simulink model "bmgen_array_N8"  (R2014a)
settings: Solver=ode45  StartTime=0.0  StopTime=Tmax  RelTol=1e-3
values from neighbouring files (symbols this model uses):
  Tgrid = (1 / Fgrid)    (= 0.0166666666667)    [array_init.m]
  Ts = Tthd    (= 1.66666666667e-05)    [array_init.m]
  Tstartup = 3e-3    (= 0.003)    [array_init.m]
  Vgrid = (sqrt(2)*Vgridrms)    [array_init.m]
undefined symbols (not defined in the file or in its folder): Acarray, Aoarray, Bcarray, Boarray, Carray, Darray, Larray, N, Rarray, TswitchArray
libraries: module_switch x8, powerlib_meascontrol x3
settings Model: Creator=Taylor  LastModifiedBy=Taylor

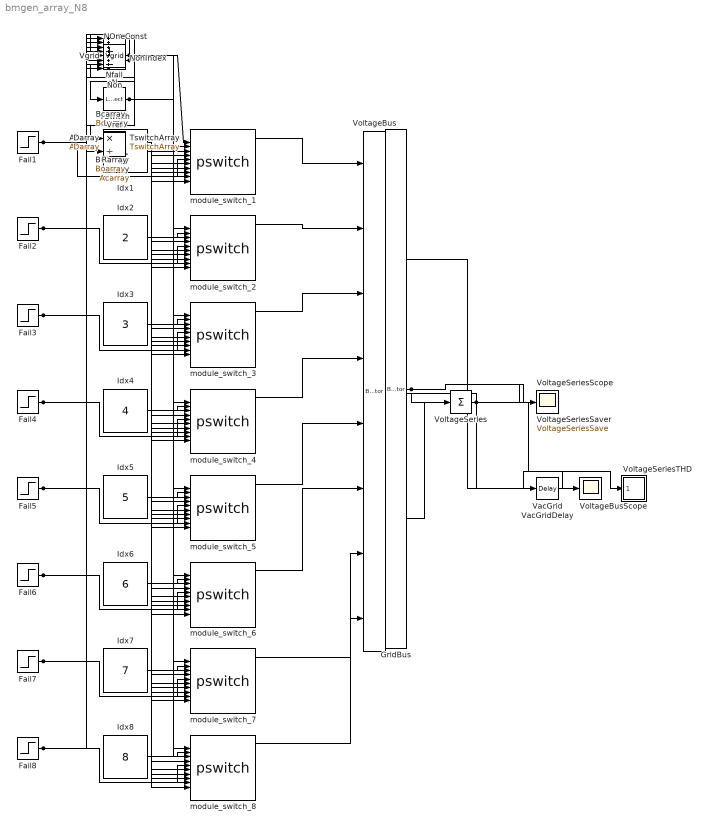
== system bmgen_array_N8 ==
  Acarray : Constant  Value=Acarray
  Aoarray : Constant  Value=Aoarray
  Bcarray : Constant  Value=Bcarray
  Boarray : Constant  Value=Boarray
  Carray : Constant  Value=Carray
  Darray : Constant  Value=Darray
  Fail{1..8} (8 alike) : Step  Time=0  After=0
  GridBus : BusCreator  Inputs=2
  Idx1 : Constant
  Idx2 : Constant  Value=2
  Idx3 : Constant  Value=3
  Idx4 : Constant  Value=4
  Idx5 : Constant  Value=5
  Idx6 : Constant  Value=6
  Idx7 : Constant  Value=7
  Idx8 : Constant  Value=8
  Larray : Constant  Value=Larray
  N : Constant  Value=N
  NOneConst : Constant
  Nfail : Sum  Inputs=++++++++  SaturateOnIntegerOverflow=on  InputSameDT=on  OutDataTypeStr=Inherit: Same as first input
  Non : Sum  Inputs=+-  SaturateOnIntegerOverflow=on  InputSameDT=on  OutDataTypeStr=Inherit: Same as first input
  NonIndex : Sum  Inputs=+-  SaturateOnIntegerOverflow=on  InputSameDT=on  OutDataTypeStr=Inherit: Same as first input
  Rarray : Constant  Value=Rarray
  TSwitch : LookupNDDirect  NumberOfTableDimensions=3  InputsSelectThisObjectFromTable=2-D Matrix  Table=TswitchArray
  TswitchArray : Constant  Value=TswitchArray
  VacGrid : Sin  Amplitude=Vgrid  Frequency=2*pi/Tgrid
  VacGridDelay : TransportDelay  DelayTime=Tstartup
  Vgrid : Constant  Value=Vgrid
  VoltageBus : BusCreator  Inputs=N
  VoltageBusScope : Scope
  VoltageSeries : Sum  Inputs=+  SaturateOnIntegerOverflow=on  InputSameDT=on  OutDataTypeStr=Inherit: Same as first input
  VoltageSeriesSaver : ToWorkspace  VariableName=VoltageSeriesSave
  VoltageSeriesScope : Scope
      settings: SaveName=ScopeDataSeries
  VoltageSeriesTHD : Subsystem  VariantControl=Variant1
  Vref : Product  Inputs=*/  SaturateOnIntegerOverflow=on  RndMeth=Zero  InputSameDT=on  OutDataTypeStr=Inherit: Same as first input
  module_switch_{1..8} (8 alike) : module_switch/pswitch
  wires:
  VacGrid/1 -> VacGridDelay/1
  VacGridDelay/1 -> GridBus/1
  N/1 -> Non/1, module_switch_1/1, module_switch_2/1, module_switch_3/1, module_switch_4/1, module_switch_5/1, module_switch_6/1, module_switch_7/1, module_switch_8/1
  Nfail/1 -> Non/2
  Non/1 -> NonIndex/1, Vref/2
  NOneConst/1 -> NonIndex/2
  Vgrid/1 -> Vref/1
  NonIndex/1 -> TSwitch/1
  VoltageSeries/1 -> GridBus/2, VoltageSeriesTHD/1(In1)
  VoltageBus/1 -> VoltageSeries/1, VoltageBusScope/1
  GridBus/1 -> VoltageSeriesScope/1, VoltageSeriesSaver/1
  Idx1/1 -> module_switch_1/2
  Fail1/1 -> module_switch_1/5, Nfail/1
  TSwitch/1 -> module_switch_1/3, module_switch_2/3, module_switch_3/3, module_switch_4/3, module_switch_5/3, module_switch_6/3, module_switch_7/3, module_switch_8/3
  Darray/1 -> module_switch_1/4, module_switch_2/4, module_switch_3/4, module_switch_4/4, module_switch_5/4, module_switch_6/4, module_switch_7/4, module_switch_8/4
  Acarray/1 -> module_switch_1/6, module_switch_2/6, module_switch_3/6, module_switch_4/6, module_switch_5/6, module_switch_6/6, module_switch_7/6, module_switch_8/6
  Aoarray/1 -> module_switch_1/7, module_switch_2/7, module_switch_3/7, module_switch_4/7, module_switch_5/7, module_switch_6/7, module_switch_7/7, module_switch_8/7
  Bcarray/1 -> module_switch_1/9, module_switch_2/9, module_switch_3/9, module_switch_4/9, module_switch_5/9, module_switch_6/9, module_switch_7/9, module_switch_8/9
  Boarray/1 -> module_switch_1/8, module_switch_2/8, module_switch_3/8, module_switch_4/8, module_switch_5/8, module_switch_6/8, module_switch_7/8, module_switch_8/8
  Vref/1 -> module_switch_1/10, module_switch_2/10, module_switch_3/10, module_switch_4/10, module_switch_5/10, module_switch_6/10, module_switch_7/10, module_switch_8/10
  module_switch_1/1 -> VoltageBus/1
  Idx2/1 -> module_switch_2/2
  Fail2/1 -> module_switch_2/5, Nfail/2
  module_switch_2/1 -> VoltageBus/2
  Idx3/1 -> module_switch_3/2
  Fail3/1 -> module_switch_3/5, Nfail/3
  module_switch_3/1 -> VoltageBus/3
  Idx4/1 -> module_switch_4/2
  Fail4/1 -> module_switch_4/5, Nfail/4
  module_switch_4/1 -> VoltageBus/4
  Idx5/1 -> module_switch_5/2
  Fail5/1 -> module_switch_5/5, Nfail/5
  module_switch_5/1 -> VoltageBus/5
  Idx6/1 -> module_switch_6/2
  Fail6/1 -> module_switch_6/5, Nfail/6
  module_switch_6/1 -> VoltageBus/6
  Idx7/1 -> module_switch_7/2
  Fail7/1 -> module_switch_7/5, Nfail/7
  module_switch_7/1 -> VoltageBus/7
  Idx8/1 -> module_switch_8/2
  Fail8/1 -> module_switch_8/5, Nfail/8
  module_switch_8/1 -> VoltageBus/8

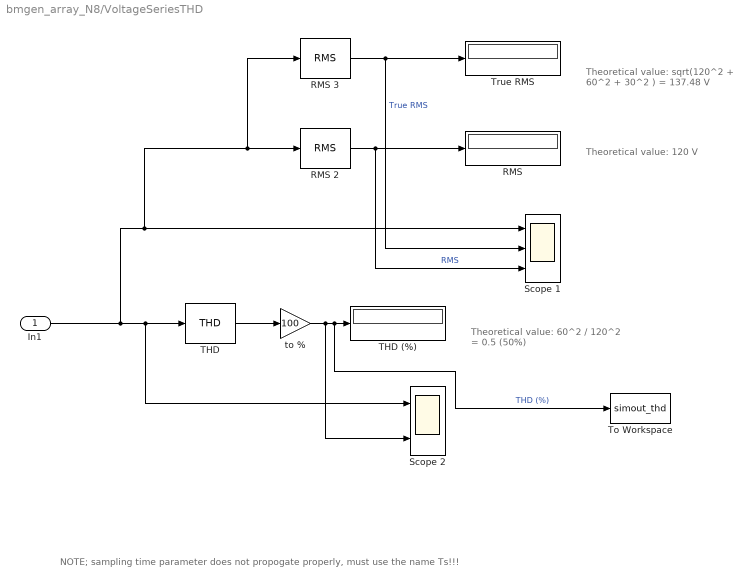
== system bmgen_array_N8/VoltageSeriesTHD ==
  note: NOTE; sampling time parameter does not propogate properly, must use the name Ts!!!
  note: Theoretical value:
      | 60^2 / 120^2 = 0.5  (50%)
  note: Theoretical value:
      | sqrt(120^2 + 60^2 + 30^2 )
      | = 137.48 V
  note: Theoretical value:
      | 120 V
  In1 : Inport
  RMS : Display
      settings: Format=bank
  RMS 2 : powerlib_meascontrol/Measurements/RMS  TrueRMS=off  Freq=Fgrid  RMSInit=Vgridrms  Ts=Ts
  RMS 3 : powerlib_meascontrol/Measurements/RMS  TrueRMS=on  Freq=Fgrid  RMSInit=Vgridrms  Ts=Ts
  Scope 1 : Scope  NumInputPorts=3
      settings: TimeRange=0.1  YMin=-250~50~50  YMax=250~150~150  SaveName=ScopeData2
  Scope 2 : Scope  NumInputPorts=2
      settings: TimeRange=0.0333333  YMin=-550~0  YMax=500~50
  THD : powerlib_meascontrol/Measurements/THD  Freq=Fgrid  Ts=Ts
  THD (%) : Display
      settings: Format=bank
  To Workspace : ToWorkspace  VariableName=simout_thd  SaveFormat=Timeseries  SampleTime=-1
  True RMS : Display
      settings: Format=bank
  to % : Gain  Gain=100  SampleTime=Ts
  wires:
  THD/1 -> to %/1
  to %/1 -> THD (%)/1, To Workspace/1, Scope 2/2  "THD (%)"
  In1/1 -> RMS 2/1, RMS 3/1, Scope 1/1, Scope 2/1, THD/1
  RMS 2/1 -> RMS/1, Scope 1/3  "RMS"
  RMS 3/1 -> True RMS/1, Scope 1/2  "True RMS"
